simulink model "two_vehicle"  (R2020a)
settings: Solver=ode3  StartTime=0.0  StopTime=90  FixedStep=0.02  RelTol=1e-3  EnableMultiTasking=on
undefined symbols (not defined in the file): control, data
libraries: simulink_need_slupdate x10, simulink x2
settings Model: SimulationMode=accelerator  Creator=Owen  LastModifiedBy=rangeesh
settings DataIOCC: LimitDataPoints=on  SaveFormat=Array  ReturnWorkspaceOutputs=off
settings OptimizationCC: LifeSpan=inf  AccelVerboseBuild=on
settings DebuggingCC: SolverPrmCheckMsg=warning  SFUnexpectedBacktrackingDiag=warning  SFNoUnconditionalDefaultTransitionDiag=warning  SFExecutionAtInitializationDiag=none  ArithmeticOperatorsInVariantConditions=warning
settings HardwareCC: ProdBitPerPointer=32  ProdBitPerSizeT=32  ProdBitPerPtrDiffT=32  ProdLargestAtomicFloat=None  ProdIntDivRoundTo=Undefined  ProdEndianess=Unspecified  ProdWordSize=32  ProdHWDeviceType=32-bit Generic
settings ModelReferenceCC: PropagateSignalLabelsOutOfModel=off
settings SFSimCC: SimCustomInitializer=initTORCSLink();  SimCustomTerminator=terminateTORCSLink();  SimUserSources=TORCSLink.c  SimUserLibraries=librt.so  SimUseLocalCustomCode=off  SimParseCustomCode=off  SimBuildMode=sf_nonincremental_build  SimGenImportedTypeDefs=on  CustomCodeUndefinedFunction=UseInterfaceOnly
settings RTWCC: RTWUseLocalCustomCode=off
settings CodeAppCC: StateflowObjectComments=on
settings GRTTargetCC: TargetLangStandard=C89/C90 (ANSI)
settings ConfigComp: CovMetricSettings=dw  CovHtmlReporting=on  CovSaveCumulativeToWorkspaceVar=on  CovSaveSingleToWorkspaceVar=on  CovExternalEMLEnable=off  CovSFcnEnable=off

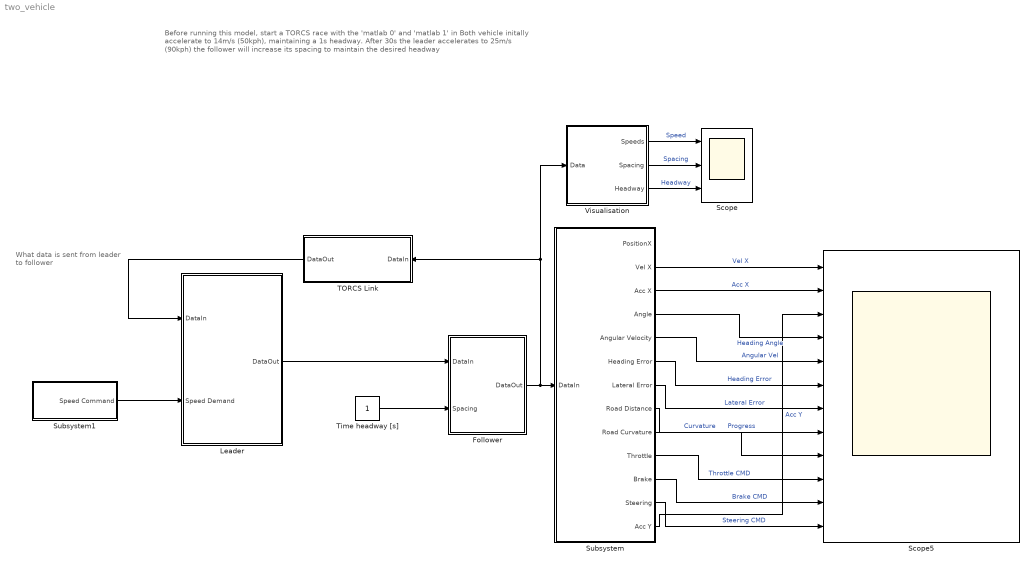
== system two_vehicle ==
  note: What data is sent from leader to follower
  note: Before running this model, start a TORCS race with the 'matlab 0' and 'matlab 1' in
      |
      | Both vehicle initally accelerate to 14m/s (50kph), maintaining a 1s headway.
      | After 30s the leader accelerates to 25m/s (90kph)
      | the follower will increase its spacing to maintain the desired headway
  Follower : Subsystem
      settings: CopyFcn=|
      | veh = str2num(get_param(gcb, 'vehicle'));
      | veh = veh + 1;
      | set_param(gcb,'vehicle',num2str(veh));
  Leader : Subsystem
  Scope : Scope  NumInputPorts=3
  Scope5 : Scope  NumInputPorts=12
  Subsystem : Subsystem
  Subsystem1 : Subsystem
  TORCS Link : Subsystem  LoadFcn=|  InitFcn=|
      LoadFcn=|
      | load VehicleBusses.mat;
      | src = 'TORCSLink.c';
      | init = 'initTORCSLink();';
      | term = 'terminateTORCSLink();';
      | simSrc = get_param(gcs,'SimUserSources');
      | simInit = get_param(gcs,'SimCustomInitializer');
      | simTerm = get_param(gcs,'SimCustomTerminator');
      | 
      | if isempty(strfind(simSrc,src))
      |   fprintf('Adding %s to Custom Sources\n', src);
      |   set_param(gcs,'SimUserSources', [simSrc 10 src]);
      | end
      | 
      | if isempty(strfind(simInit,init))
      |   fprintf('Adding %s to Custom Initialisation Code\n', init);
      |   set_param(gcs,'SimCustomInitializer', [simInit 10 init]);
      | end
      | 
      | if isempty(strfind(simTerm,term))
      |   fprintf('Adding %s to Custom Termination Code\n', term);
      |   set_param(gcs,'SimCustomTerminator', [simTerm 10 term]);
      | end
      | 
      | if isunix
      |     libs = 'librt.so';
      |     simLibs = get_param(gcs,'SimUserLibraries');
      | 
      |     if isempty(strfind(simLibs,libs))
      |       fprintf('Adding %s to Custom Libraries\n', libs);
      |       set_param(gcs,'SimUserLibraries', [simLibs 10 libs]);
      |     end
      | else
      |    set_param(gcs,'SimUserLibraries', '');
      | end
      | 
      | clear src init term simSrc simInit simTerm libs simLibs;
      InitFcn=|
      | load VehicleBusses.mat;
      | src = 'TORCSLink.c';
      | init = 'initTORCSLink();';
      | term = 'terminateTORCSLink();';
      | simSrc = get_param(gcs,'SimUserSources');
      | simInit = get_param(gcs,'SimCustomInitializer');
      | simTerm = get_param(gcs,'SimCustomTerminator');
      | 
      | if isempty(strfind(simSrc,src))
      |   fprintf('Adding %s to Custom Sources\n', src);
      |   set_param(gcs,'SimUserSources', [simSrc 10 src]);
      | end
      | 
      | if isempty(strfind(simInit,init))
      |   fprintf('Adding %s to Custom Initialisation Code\n', init);
      |   set_param(gcs,'SimCustomInitializer', [simInit 10 init]);
      | end
      | 
      | if isempty(strfind(simTerm,term))
      |   fprintf('Adding %s to Custom Termination Code\n', term);
      |   set_param(gcs,'SimCustomTerminator', [simTerm 10 term]);
      | end
      | 
      | if isunix
      |     libs = 'librt.so';
      |     simLibs = get_param(gcs,'SimUserLibraries');
      | 
      |     if isempty(strfind(simLibs,libs))
      |       fprintf('Adding %s to Custom Libraries\n', libs);
      |       set_param(gcs,'SimUserLibraries', [simLibs 10 libs]);
      |     end
      | else
      |    set_param(gcs,'SimUserLibraries', '');
      | end
      | 
      | clear src init term simSrc simInit simTerm libs simLibs;
  Time headway [s] : Constant
  Visualisation : Subsystem
  wires:
  Follower/1(DataOut) -> Visualisation/1(Data), TORCS Link/1(DataIn), Subsystem/1(DataIn)
  Leader/1(DataOut) -> Follower/1(DataIn)
  Time headway [s]/1 -> Follower/2(Spacing)
  Subsystem1/1(Speed Command) -> Leader/2(Speed Demand)
  Visualisation/2(Spacing) -> Scope/2  "Spacing"
  Visualisation/3(Headway) -> Scope/3  "Headway"
  Subsystem/2(Vel X) -> Scope5/1  "Vel X"
  Subsystem/3(Acc X) -> Scope5/2  "Acc X"
  Subsystem/11(Brake) -> Scope5/11  "Brake CMD"
  Subsystem/5(Angular Velocity) -> Scope5/5  "Angular Vel"
  Subsystem/10(Throttle) -> Scope5/10  "Throttle CMD"
  Visualisation/1(Speeds) -> Scope/1  "Speed"
  TORCS Link/1(DataOut) -> Leader/1(DataIn)
  Subsystem/12(Steering) -> Scope5/12  "Steering CMD"
  Subsystem/9(Road Curvature) -> Scope5/9  "Curvature"
  Subsystem/8(Road Distance) -> Scope5/8  "Progress"
  Subsystem/7(Lateral Error) -> Scope5/7  "Lateral Error"
  Subsystem/4(Angle) -> Scope5/4  "Heading Angle"
  Subsystem/6(Heading Error) -> Scope5/6  "Heading Error"
  Subsystem/13(Acc Y) -> Scope5/3  "Acc Y"

== system two_vehicle/Follower ==
  note: Use a Selector block to choose which vehicle data you want,
      | then use an Assignment to overwrite that vehicles data when you're done...
  DataIn : Inport
  Spacing : Inport  Port=2
  Assignment : Assignment  DiagnosticForDimensions=Warning  IndexOptions=Index vector (dialog)  Indices=2  OutputSizes=1
  Ego : Selector  InputPortWidth=10  IndexOptions=Index vector (dialog)  Indices=2  OutputSizes=1
  Follower Vehicle Control : Subsystem
  Leader : Selector  InputPortWidth=10  IndexOptions=Index vector (dialog)  Indices=1  OutputSizes=1
  DataOut : Outport
  wires:
  Ego/1 -> Follower Vehicle Control/3(Ego)
  DataIn/1 -> Ego/1, Leader/1, Assignment/1
  Assignment/1 -> DataOut/1
  Spacing/1 -> Follower Vehicle Control/1(Headway)
  Follower Vehicle Control/1(Data Out) -> Assignment/2
  Leader/1 -> Follower Vehicle Control/2(Leader)

== system two_vehicle/Leader ==
  note: Selector block is there to select which vehicle's
      | data you want to send
  note: Use a Selector block to choose which vehicle data you want,
      | then use an Assignment to overwrite that vehicles data when you're done...
  DataIn : Inport
  Speed Demand : Inport  Port=2
  Assignment : Assignment  DiagnosticForDimensions=Warning  IndexOptions=Index vector (dialog)  Indices=1  OutputSizes=1
  Lead Vehicle Control : Subsystem
  Selector : Selector  InputPortWidth=10  IndexOptions=Index vector (dialog)  Indices=1  OutputSizes=1
  DataOut : Outport
  wires:
  Speed Demand/1 -> Lead Vehicle Control/2(Speed Demand)
  DataIn/1 -> Selector/1, Assignment/1
  Selector/1 -> Lead Vehicle Control/1(Data In)
  Assignment/1 -> DataOut/1
  Lead Vehicle Control/1(Data Out) -> Assignment/2

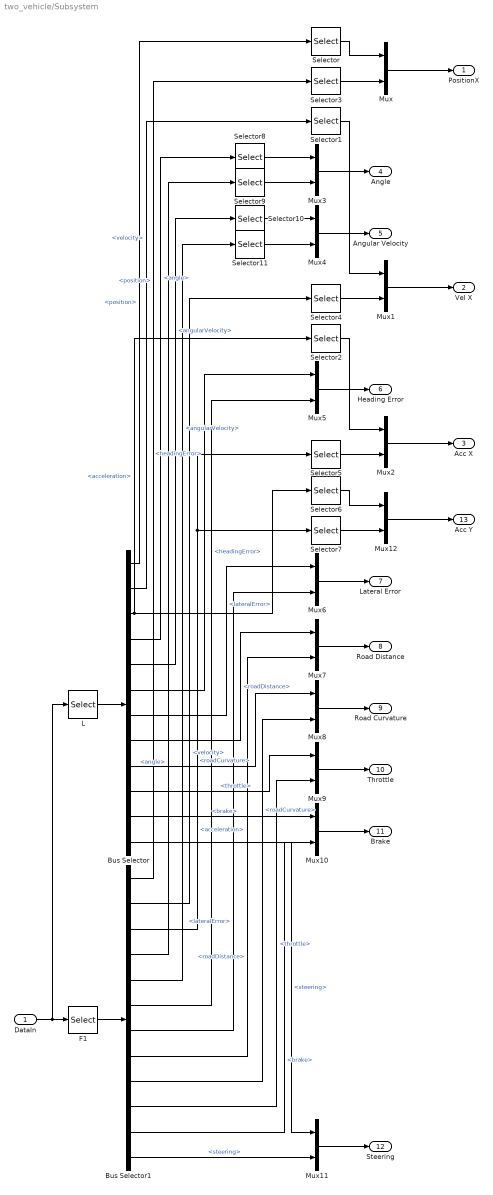
== system two_vehicle/Subsystem ==
  DataIn : Inport
  Bus Selector : BusSelector  OutputSignals=data.position,data.velocity,data.acceleration,data.angle,data.angularVelocity,data.headingError,data.lateralError,data.roadDistance,data.roadCurvature,control.throttle,control.brake,control.steering
  Bus Selector1 : BusSelector  OutputSignals=data.position,data.velocity,data.acceleration,data.angle,data.angularVelocity,data.headingError,data.lateralError,data.roadDistance,data.roadCurvature,control.throttle,control.brake,control.steering
  F1 : Selector  InputPortWidth=10  IndexOptions=Index vector (dialog)  Indices=2  OutputSizes=1
  L : Selector  InputPortWidth=10  IndexOptions=Index vector (dialog)  Indices=1  OutputSizes=1
  Mux{,1..12} (13 alike) : Mux  Inputs=2
  Selector{,1..5} (6 alike) : Selector  InputPortWidth=3  IndexOptions=Index vector (dialog)  Indices=1  OutputSizes=1
  Selector{8..11} (4 alike) : Selector  InputPortWidth=3  IndexOptions=Index vector (dialog)  Indices=3  OutputSizes=1
  Selector6 : Selector  InputPortWidth=3  IndexOptions=Index vector (dialog)  Indices=2  OutputSizes=1
  Selector7 : Selector  InputPortWidth=3  IndexOptions=Index vector (dialog)  Indices=2  OutputSizes=1
  PositionX : Outport
  Vel X : Outport  Port=2
  Acc X : Outport  Port=3
  Angle : Outport  Port=4
  Angular Velocity : Outport  Port=5
  Heading Error : Outport  Port=6
  Lateral Error : Outport  Port=7
  Road Distance : Outport  Port=8
  Road Curvature : Outport  Port=9
  Throttle : Outport  Port=10
  Brake : Outport  Port=11
  Steering : Outport  Port=12
  Acc Y : Outport  Port=13
  wires:
  Bus Selector/3 -> Selector6/1, Selector2/1  "<acceleration>"
  DataIn/1 -> F1/1, L/1
  Selector6/1 -> Mux12/1
  Mux7/1 -> Road Distance/1
  Bus Selector/11 -> Mux10/1  "<brake>"
  Bus Selector/6 -> Mux5/1  "<headingError>"
  Bus Selector/4 -> Selector8/1  "<angle>"
  Bus Selector/5 -> Selector10/1  "<angularVelocity>"
  Bus Selector1/5 -> Selector11/1  "<angularVelocity>"
  Mux4/1 -> Angular Velocity/1
  Mux9/1 -> Throttle/1
  Mux1/1 -> Vel X/1
  Mux6/1 -> Lateral Error/1
  Bus Selector1/7 -> Mux6/2  "<lateralError>"
  Selector/1 -> Mux/1
  Bus Selector1/3 -> Selector7/1, Selector5/1  "<acceleration>"
  Bus Selector1/12 -> Mux11/2  "<steering>"
  Selector3/1 -> Mux/2
  Selector4/1 -> Mux1/2
  Mux5/1 -> Heading Error/1
  Mux10/1 -> Brake/1
  Bus Selector1/9 -> Mux8/2  "<roadCurvature>"
  Mux8/1 -> Road Curvature/1
  Bus Selector/12 -> Mux11/1  "<steering>"
  F1/1 -> Bus Selector1/1
  Bus Selector1/10 -> Mux9/2  "<throttle>"
  Mux/1 -> PositionX/1
  Mux11/1 -> Steering/1
  Bus Selector1/11 -> Mux10/2  "<brake>"
  Bus Selector/10 -> Mux9/1  "<throttle>"
  Bus Selector/7 -> Mux6/1  "<lateralError>"
  Bus Selector/9 -> Mux8/1  "<roadCurvature>"
  Bus Selector1/2 -> Selector4/1  "<velocity>"
  Bus Selector1/1 -> Selector3/1  "<position>"
  Mux12/1 -> Acc Y/1
  Bus Selector1/4 -> Selector9/1  "<angle>"
  Bus Selector1/6 -> Mux5/2  "<headingError>"
  Selector7/1 -> Mux12/2
  Selector2/1 -> Mux2/1
  L/1 -> Bus Selector/1
  Bus Selector/2 -> Selector1/1  "<velocity>"
  Selector1/1 -> Mux1/1
  Bus Selector1/8 -> Mux7/2  "<roadDistance>"
  Mux2/1 -> Acc X/1
  Bus Selector/1 -> Selector/1  "<position>"
  Bus Selector/8 -> Mux7/1  "<roadDistance>"
  Selector5/1 -> Mux2/2
  Mux3/1 -> Angle/1
  Selector8/1 -> Mux3/1
  Selector9/1 -> Mux3/2
  Selector10/1 -> Mux4/1
  Selector11/1 -> Mux4/2

== system two_vehicle/Subsystem1 ==
  Clock : Clock
  Constant : Constant  Value=[14, 25, 0]
  Index Selector : MATLAB Function  TreatAsAtomicUnit=on
  Selector : Selector  InputPortWidth=3  IndexOptions=Index vector (port)  Indices=[1 3]  OutputSizes=1
  Speed Command : Outport
  wires:
  Clock/1 -> Index Selector/1(time)
  Index Selector/1(speed_command_index) -> Selector/2
  Constant/1 -> Selector/1
  Selector/1 -> Speed Command/1

== system two_vehicle/TORCS Link ==
  note: This subsystem handles the communicatrion with TORCS via a MATLAB function.
      | The simulation must be configured to run at a fixed sample time equal to the rate at which TORCS updates its robots (0.02s by default)
      | Data returned from TORCS is passed through a First-Order-Hold to allow continuous design in Simulink
      | Data for a maximum of 10 vehicles is returned, but not all vehicles need be present in the race
  DataIn : Inport
  FOHs : Subsystem  TreatAsAtomicUnit=on
  Memory : Memory
  Stop Simulation : Stop
  TORCSLink : MATLAB Function  TreatAsAtomicUnit=on
  DataOut : Outport
  wires:
  Memory/1 -> TORCSLink/1(vehicleDataIn)
  TORCSLink/1(vehicleDataOut) -> FOHs/1(In1)
  FOHs/1(Out1) -> DataOut/1
  DataIn/1 -> Memory/1
  TORCSLink/2(stop) -> Stop Simulation/1

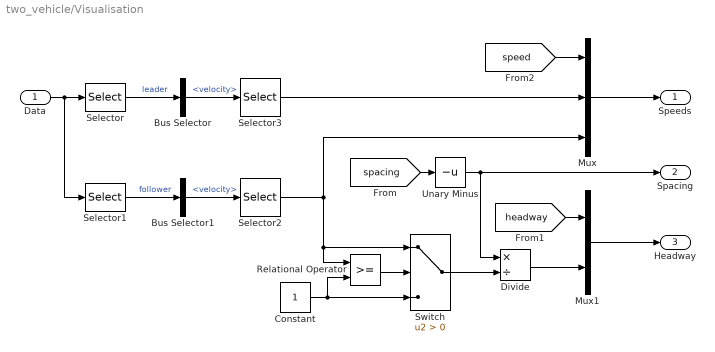
== system two_vehicle/Visualisation ==
  Data : Inport
  Bus Selector : BusSelector  OutputSignals=data.velocity
  Bus Selector1 : BusSelector  OutputSignals=data.velocity
  Constant : Constant
  Divide : Product  Inputs=*/
  Mux : Mux  Inputs=3
  Mux1 : Mux  Inputs=2
  Relational Operator : RelationalOperator  OutDataTypeStr=boolean  RndMeth=Nearest
  Selector : Selector  InputPortWidth=10  IndexOptions=Index vector (dialog)  Indices=1  OutputSizes=1
  Selector1 : Selector  InputPortWidth=10  IndexOptions=Index vector (dialog)  Indices=2  OutputSizes=1
  Selector2 : Selector  InputPortWidth=3  IndexOptions=Index vector (dialog)  Indices=1  OutputSizes=1
  Selector3 : Selector  InputPortWidth=3  IndexOptions=Index vector (dialog)  Indices=1  OutputSizes=1
  Switch : Switch  Criteria=u2 > Threshold
  Unary Minus : UnaryMinus
  Speeds : Outport
  Spacing : Outport  Port=2
  Headway : Outport  Port=3
  wires:
  Data/1 -> Selector1/1, Selector/1
  Selector/1 -> Bus Selector/1  "leader"
  Selector1/1 -> Bus Selector1/1  "follower"
  Bus Selector1/1 -> Selector2/1  "<velocity>"
  Bus Selector/1 -> Selector3/1  "<velocity>"
  Selector3/1 -> Mux/2
  Selector2/1 -> Relational Operator/1, Switch/1, Mux/3
  Mux/1 -> Speeds/1
  [spacing] -> Unary Minus/1
  Unary Minus/1 -> Divide/1, Spacing/1
  [speed] -> Mux/1
  Mux1/1 -> Headway/1
  Divide/1 -> Mux1/2
  [headway] -> Mux1/1
  Switch/1 -> Divide/2
  Relational Operator/1 -> Switch/2
  Constant/1 -> Switch/3, Relational Operator/2

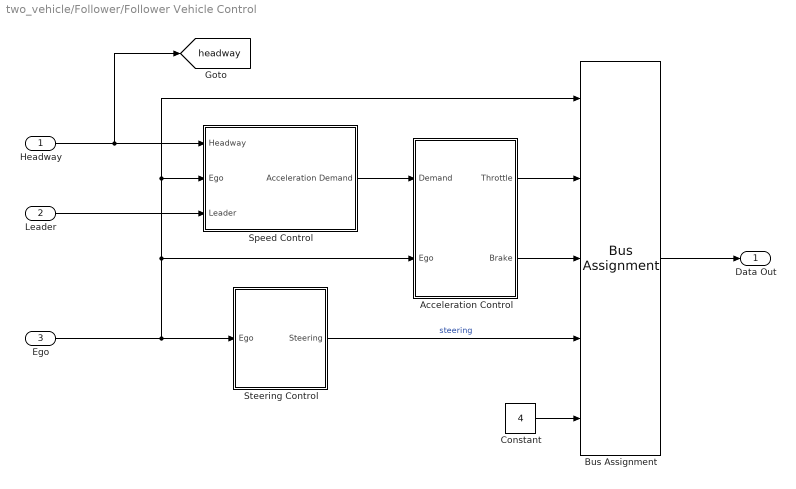
== system two_vehicle/Follower/Follower Vehicle Control ==
  Headway : Inport
  Leader : Inport  Port=2
  Ego : Inport  Port=3
  Acceleration Control : Subsystem
  Bus Assignment : BusAssignment  AssignedSignals=control.throttle,control.brake,control.steering,control.gear
  Constant : Constant  Value=4  OutDataTypeStr=int32
  Speed Control : Subsystem
  Steering Control : Subsystem
  Data Out : Outport
  tag scope: headway=global
  wires:
  Bus Assignment/1 -> Data Out/1
  Speed Control/1(Acceleration Demand) -> Acceleration Control/1(Demand)
  Headway/1 -> [headway], Speed Control/1(Headway)
  Ego/1 -> Bus Assignment/1, Speed Control/2(Ego), Acceleration Control/2(Ego), Steering Control/1(Ego)
  Leader/1 -> Speed Control/3(Leader)
  Acceleration Control/2(Brake) -> Bus Assignment/3
  Acceleration Control/1(Throttle) -> Bus Assignment/2
  Steering Control/1(Steering) -> Bus Assignment/4  "steering"
  Constant/1 -> Bus Assignment/5

== system two_vehicle/Leader/Lead Vehicle Control ==
  Data In : Inport
  Speed Demand : Inport  Port=2
  Acceleration Control : Subsystem
  Bus Assignment : BusAssignment  AssignedSignals=control.throttle,control.brake,control.steering,control.gear
  Constant : Constant  Value=4  OutDataTypeStr=int32
  Speed Control : Subsystem
  Steering Control : Subsystem
  Data Out : Outport
  tag scope: speed=global
  wires:
  Speed Demand/1 -> [speed], Speed Control/1(Demand)
  Bus Assignment/1 -> Data Out/1
  Speed Control/1(Acceleration Demand) -> Acceleration Control/1(Demand)
  Data In/1 -> Steering Control/1(Ego), Speed Control/2(Velocity), Bus Assignment/1, Acceleration Control/2(Ego)
  Acceleration Control/2(Brake) -> Bus Assignment/3
  Acceleration Control/1(Throttle) -> Bus Assignment/2
  Steering Control/1(Steering) -> Bus Assignment/4
  Constant/1 -> Bus Assignment/5

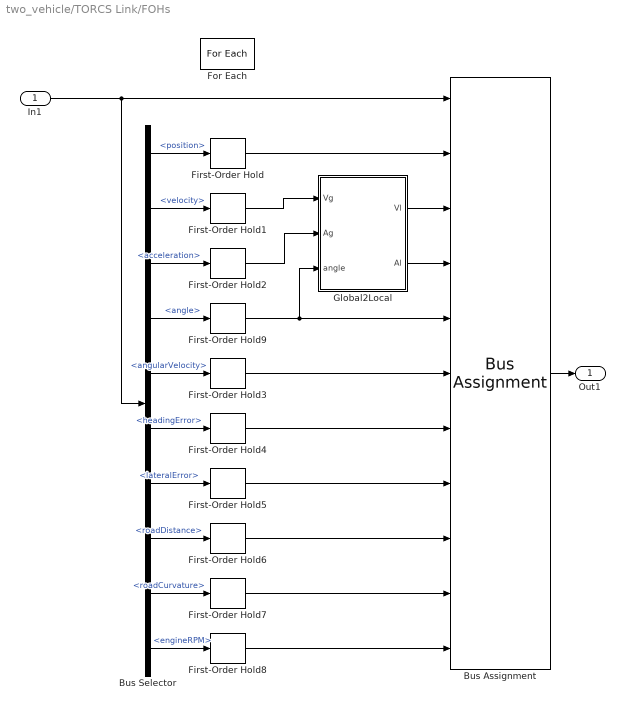
== system two_vehicle/TORCS Link/FOHs ==
  In1 : Inport  Partition=on  PartitionDimension=1  PartitionWidth=1  PartitionOffset=0
  Bus Assignment : BusAssignment  AssignedSignals=data.position,data.velocity,data.acceleration,data.angle,data.angularVelocity,data.headingError,data.lateralError,data.roadDistance,data.roadCurvature,data.engineRPM
  Bus Selector : BusSelector  OutputSignals=data.position,data.velocity,data.acceleration,data.angle,data.angularVelocity,data.headingError,data.lateralError,data.roadDistance,data.roadCurvature,data.engineRPM
  First-Order Hold{,1..9} (10 alike) : simulink_need_slupdate/First-Order Hold  DisableCoverage=on  Ts=0.02
      settings: SourceProductBaseCode=SL
  For Each : ForEach  DisableCoverage=on
  Global2Local : MATLAB Function  TreatAsAtomicUnit=on
  Out1 : Outport  ConcatenationDimension=1
  wires:
  Bus Assignment/1 -> Out1/1
  Bus Selector/10 -> First-Order Hold8/1  "<engineRPM>"
  Bus Selector/9 -> First-Order Hold7/1  "<roadCurvature>"
  Bus Selector/8 -> First-Order Hold6/1  "<roadDistance>"
  Bus Selector/7 -> First-Order Hold5/1  "<lateralError>"
  Bus Selector/6 -> First-Order Hold4/1  "<headingError>"
  Bus Selector/5 -> First-Order Hold3/1  "<angularVelocity>"
  Bus Selector/3 -> First-Order Hold2/1  "<acceleration>"
  Bus Selector/2 -> First-Order Hold1/1  "<velocity>"
  Bus Selector/1 -> First-Order Hold/1  "<position>"
  In1/1 -> Bus Assignment/1, Bus Selector/1
  Bus Selector/4 -> First-Order Hold9/1  "<angle>"
  First-Order Hold9/1 -> Global2Local/3(angle), Bus Assignment/5
  First-Order Hold3/1 -> Bus Assignment/6
  First-Order Hold4/1 -> Bus Assignment/7
  First-Order Hold5/1 -> Bus Assignment/8
  First-Order Hold6/1 -> Bus Assignment/9
  First-Order Hold7/1 -> Bus Assignment/10
  First-Order Hold8/1 -> Bus Assignment/11
  First-Order Hold1/1 -> Global2Local/1(Vg)
  First-Order Hold2/1 -> Global2Local/2(Ag)
  First-Order Hold/1 -> Bus Assignment/2
  Global2Local/2(Al) -> Bus Assignment/4
  Global2Local/1(Vl) -> Bus Assignment/3

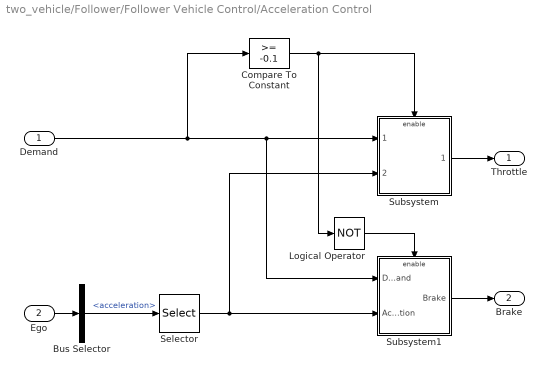
== system two_vehicle/Follower/Follower Vehicle Control/Acceleration Control ==
  Demand : Inport
  Ego : Inport  Port=2
  Bus Selector : BusSelector  OutputSignals=data.acceleration
  Compare To Constant : simulink/Logic and Bit Operations/Compare To Constant  relop=>=  const=-0.1  OutDataTypeStr=boolean
  Logical Operator : Logic  Operator=NOT  AllPortsSameDT=off  OutDataTypeStr=boolean
  Selector : Selector  InputPortWidth=3  IndexOptions=Index vector (dialog)  Indices=1  OutputSizes=1
  Subsystem : Subsystem
  Subsystem1 : Subsystem
  Throttle : Outport
  Brake : Outport  Port=2
  wires:
  Selector/1 -> Subsystem/2(Acceleration), Subsystem1/2(Acceleration)
  Demand/1 -> Compare To Constant/1, Subsystem1/1(Demand), Subsystem/1(Demand)
  Subsystem1/1(Brake) -> Brake/1
  Subsystem/1(Throttle) -> Throttle/1
  Compare To Constant/1 -> Subsystem/Enable, Logical Operator/1
  Logical Operator/1 -> Subsystem1/Enable
  Ego/1 -> Bus Selector/1
  Bus Selector/1 -> Selector/1  "<acceleration>"

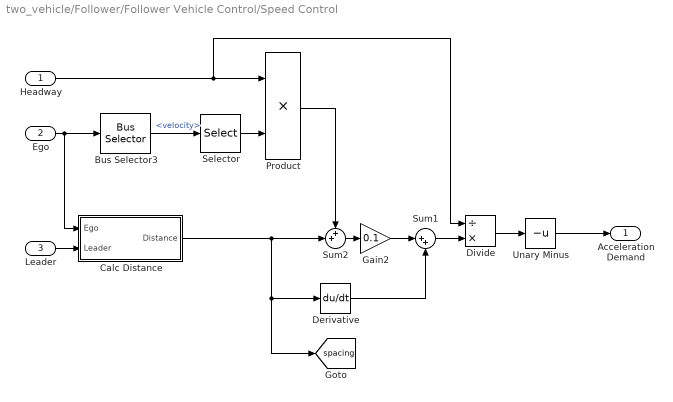
== system two_vehicle/Follower/Follower Vehicle Control/Speed Control ==
  Headway : Inport
  Ego : Inport  Port=2
  Leader : Inport  Port=3
  Bus Selector3 : BusSelector  OutputSignals=data.velocity
  Calc Distance : Subsystem
  Derivative : Derivative
  Divide : Product  Inputs=/*
  Gain2 : Gain  Gain=0.1
  Product : Product
  Selector : Selector  InputPortWidth=3  IndexOptions=Index vector (dialog)  Indices=1  OutputSizes=1
  Sum1 : Sum  Inputs=|++
  Sum2 : Sum  Inputs=++|
  Unary Minus : UnaryMinus
  Acceleration Demand : Outport
  tag scope: spacing=global
  wires:
  Ego/1 -> Calc Distance/1(Ego), Bus Selector3/1
  Leader/1 -> Calc Distance/2(Leader)
  Bus Selector3/1 -> Selector/1  "<velocity>"
  Headway/1 -> Divide/1, Product/1
  Selector/1 -> Product/2
  Calc Distance/1(Distance) -> Derivative/1, [spacing], Sum2/2
  Product/1 -> Sum2/1
  Sum2/1 -> Gain2/1
  Gain2/1 -> Sum1/1
  Derivative/1 -> Sum1/2
  Sum1/1 -> Divide/2
  Divide/1 -> Unary Minus/1
  Unary Minus/1 -> Acceleration Demand/1

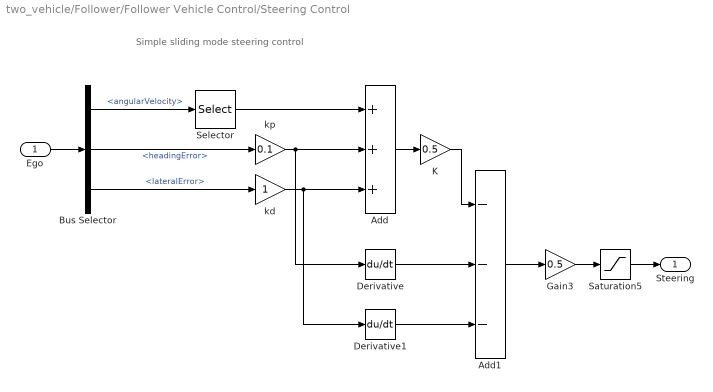
== system two_vehicle/Follower/Follower Vehicle Control/Steering Control ==
  note: Simple sliding mode steering control
  Ego : Inport
  Add : Sum  Inputs=+++
  Add1 : Sum  Inputs=---
  Bus Selector : BusSelector  OutputSignals=data.angularVelocity,data.headingError,data.lateralError
  Derivative : Derivative
  Derivative1 : Derivative
  Gain3 : Gain  Gain=0.5
  K : Gain  Gain=0.5
  Saturation5 : Saturate
  Selector : Selector  InputPortWidth=3  IndexOptions=Index vector (dialog)  Indices=3  OutputSizes=1
  kd : Gain
  kp : Gain  Gain=0.1
  Steering : Outport
  wires:
  Ego/1 -> Bus Selector/1
  Add1/1 -> Gain3/1
  K/1 -> Add1/1
  Derivative1/1 -> Add1/3
  Derivative/1 -> Add1/2
  Add/1 -> K/1
  kp/1 -> Derivative/1, Add/2
  kd/1 -> Derivative1/1, Add/3
  Bus Selector/3 -> kd/1  "<lateralError>"
  Bus Selector/2 -> kp/1  "<headingError>"
  Gain3/1 -> Saturation5/1
  Saturation5/1 -> Steering/1
  Selector/1 -> Add/1
  Bus Selector/1 -> Selector/1  "<angularVelocity>"

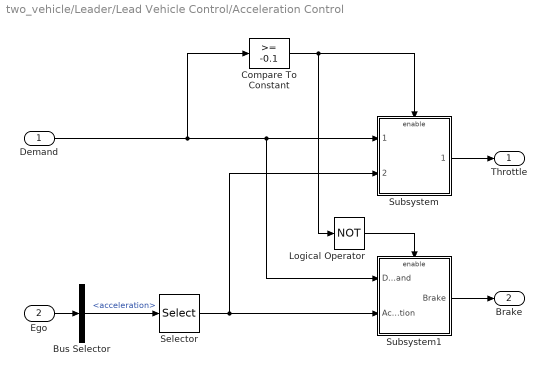
== system two_vehicle/Leader/Lead Vehicle Control/Acceleration Control ==
  Demand : Inport
  Ego : Inport  Port=2
  Bus Selector : BusSelector  OutputSignals=data.acceleration
  Compare To Constant : simulink/Logic and Bit Operations/Compare To Constant  relop=>=  const=-0.1  OutDataTypeStr=boolean
  Logical Operator : Logic  Operator=NOT  AllPortsSameDT=off  OutDataTypeStr=boolean
  Selector : Selector  InputPortWidth=3  IndexOptions=Index vector (dialog)  Indices=1  OutputSizes=1
  Subsystem : Subsystem
  Subsystem1 : Subsystem
  Throttle : Outport
  Brake : Outport  Port=2
  wires:
  Selector/1 -> Subsystem/2(Acceleration), Subsystem1/2(Acceleration)
  Demand/1 -> Compare To Constant/1, Subsystem1/1(Demand), Subsystem/1(Demand)
  Subsystem1/1(Brake) -> Brake/1
  Subsystem/1(Throttle) -> Throttle/1
  Compare To Constant/1 -> Subsystem/Enable, Logical Operator/1
  Logical Operator/1 -> Subsystem1/Enable
  Ego/1 -> Bus Selector/1
  Bus Selector/1 -> Selector/1  "<acceleration>"

== system two_vehicle/Leader/Lead Vehicle Control/Speed Control ==
  Demand : Inport
  Velocity : Inport  Port=2
  Bus Selector : BusSelector  OutputSignals=data.velocity
  Gain : Gain  Gain=0.5
  Rate Limiter : RateLimiter  RisingSlewLimit=inf  FallingSlewLimit=-inf  SampleTimeMode=inherited
  Saturation : Saturate  UpperLimit=2  LowerLimit=-4
  Selector : Selector  InputPortWidth=3  IndexOptions=Index vector (dialog)  Indices=1  OutputSizes=1
  Sum : Sum  Inputs=|+-
  Acceleration Demand : Outport
  wires:
  Gain/1 -> Saturation/1
  Sum/1 -> Gain/1
  Demand/1 -> Sum/1
  Saturation/1 -> Rate Limiter/1
  Selector/1 -> Sum/2
  Rate Limiter/1 -> Acceleration Demand/1
  Velocity/1 -> Bus Selector/1
  Bus Selector/1 -> Selector/1  "<velocity>"

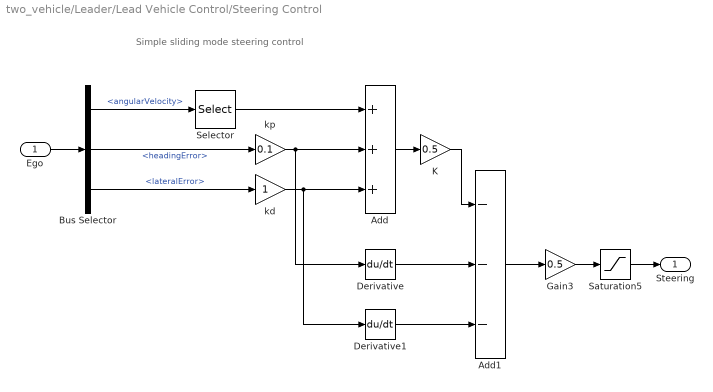
== system two_vehicle/Leader/Lead Vehicle Control/Steering Control ==
  note: Simple sliding mode steering control
  Ego : Inport
  Add : Sum  Inputs=+++
  Add1 : Sum  Inputs=---
  Bus Selector : BusSelector  OutputSignals=data.angularVelocity,data.headingError,data.lateralError
  Derivative : Derivative
  Derivative1 : Derivative
  Gain3 : Gain  Gain=0.5
  K : Gain  Gain=0.5
  Saturation5 : Saturate
  Selector : Selector  InputPortWidth=3  IndexOptions=Index vector (dialog)  Indices=3  OutputSizes=1
  kd : Gain
  kp : Gain  Gain=0.1
  Steering : Outport
  wires:
  Ego/1 -> Bus Selector/1
  Add1/1 -> Gain3/1
  K/1 -> Add1/1
  Derivative1/1 -> Add1/3
  Derivative/1 -> Add1/2
  Add/1 -> K/1
  kp/1 -> Derivative/1, Add/2
  kd/1 -> Derivative1/1, Add/3
  Bus Selector/3 -> kd/1  "<lateralError>"
  Bus Selector/2 -> kp/1  "<headingError>"
  Gain3/1 -> Saturation5/1
  Saturation5/1 -> Steering/1
  Selector/1 -> Add/1
  Bus Selector/1 -> Selector/1  "<angularVelocity>"

== system two_vehicle/Follower/Follower Vehicle Control/Acceleration Control/Subsystem ==
  Demand : Inport
  Acceleration : Inport  Port=2
  Enable : EnablePort  StatesWhenEnabling=reset
  Gain : Gain  Gain=1.5
  Gain1 : Gain  Gain=10
  Integrator Limited : Integrator  LimitOutput=on  UpperSaturationLimit=1  LowerSaturationLimit=-1
  Sum : Sum  Inputs=++|
  Sum1 : Sum  Inputs=+-|
  Throttle : Outport  OutputWhenDisabled=reset  InitialOutput=0
  wires:
  Gain/1 -> Sum/1
  Integrator Limited/1 -> Sum/2
  Gain1/1 -> Integrator Limited/1
  Sum/1 -> Throttle/1
  Demand/1 -> Sum1/1, Gain/1
  Acceleration/1 -> Sum1/2
  Sum1/1 -> Gain1/1

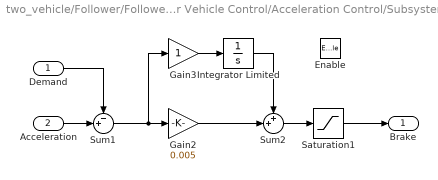
== system two_vehicle/Follower/Follower Vehicle Control/Acceleration Control/Subsystem1 ==
  Demand : Inport
  Acceleration : Inport  Port=2
  Enable : EnablePort  StatesWhenEnabling=reset
  Gain2 : Gain  Gain=0.005
  Gain3 : Gain
  Integrator Limited : Integrator  LimitOutput=on  UpperSaturationLimit=1  LowerSaturationLimit=-1
  Saturation1 : Saturate  UpperLimit=1  LowerLimit=0
  Sum1 : Sum  Inputs=-+|
  Sum2 : Sum  Inputs=++|
  Brake : Outport  OutputWhenDisabled=reset  InitialOutput=0
  wires:
  Saturation1/1 -> Brake/1
  Sum2/1 -> Saturation1/1
  Gain2/1 -> Sum2/2
  Integrator Limited/1 -> Sum2/1
  Gain3/1 -> Integrator Limited/1
  Sum1/1 -> Gain2/1, Gain3/1
  Demand/1 -> Sum1/1
  Acceleration/1 -> Sum1/2

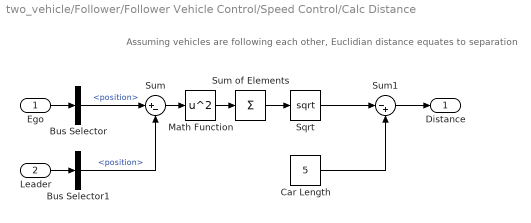
== system two_vehicle/Follower/Follower Vehicle Control/Speed Control/Calc Distance ==
  note: Assuming vehicles are following each other, Euclidian distance equates to separation
  Ego : Inport
  Leader : Inport  Port=2
  Bus Selector : BusSelector  OutputSignals=data.position
  Bus Selector1 : BusSelector  OutputSignals=data.position
  Car Length : Constant  Value=5
  Math Function : Math  Operator=square  SignedPower=on  SaturateOnIntegerOverflow=on
  Sqrt : Sqrt  SaturateOnIntegerOverflow=on
  Sum : Sum  Inputs=|+-
  Sum of Elements : Sum  Inputs=+
  Sum1 : Sum  Inputs=|-+
  Distance : Outport
  wires:
  Ego/1 -> Bus Selector/1
  Leader/1 -> Bus Selector1/1
  Bus Selector/1 -> Sum/1  "<position>"
  Bus Selector1/1 -> Sum/2  "<position>"
  Sum/1 -> Math Function/1
  Math Function/1 -> Sum of Elements/1
  Sum of Elements/1 -> Sqrt/1
  Sum1/1 -> Distance/1
  Sqrt/1 -> Sum1/1
  Car Length/1 -> Sum1/2

== system two_vehicle/Leader/Lead Vehicle Control/Acceleration Control/Subsystem ==
  note: Throttle = Demand*1.5 + Integral Error*10?
  Demand : Inport
  Acceleration : Inport  Port=2
  Enable : EnablePort  StatesWhenEnabling=reset
  Gain : Gain  Gain=1.5
  Gain1 : Gain  Gain=10
  Integrator Limited : Integrator  LimitOutput=on  UpperSaturationLimit=1  LowerSaturationLimit=-1
  Sum : Sum  Inputs=++|
  Sum1 : Sum  Inputs=+-|
  Throttle : Outport  OutputWhenDisabled=reset  InitialOutput=0
  wires:
  Gain/1 -> Sum/1
  Integrator Limited/1 -> Sum/2
  Gain1/1 -> Integrator Limited/1
  Sum/1 -> Throttle/1
  Demand/1 -> Sum1/1, Gain/1
  Acceleration/1 -> Sum1/2
  Sum1/1 -> Gain1/1

== system two_vehicle/Leader/Lead Vehicle Control/Acceleration Control/Subsystem1 ==
  note: Error*0.005 + Integral Error * 1
  Demand : Inport
  Acceleration : Inport  Port=2
  Enable : EnablePort  StatesWhenEnabling=reset
  Gain2 : Gain  Gain=0.005
  Gain3 : Gain
  Integrator Limited : Integrator  LimitOutput=on  UpperSaturationLimit=1  LowerSaturationLimit=-1
  Saturation1 : Saturate  UpperLimit=1  LowerLimit=0
  Sum1 : Sum  Inputs=-+|
  Sum2 : Sum  Inputs=++|
  Brake : Outport  OutputWhenDisabled=reset  InitialOutput=0
  wires:
  Saturation1/1 -> Brake/1
  Sum2/1 -> Saturation1/1
  Gain2/1 -> Sum2/2
  Integrator Limited/1 -> Sum2/1
  Gain3/1 -> Integrator Limited/1
  Sum1/1 -> Gain2/1, Gain3/1
  Demand/1 -> Sum1/1
  Acceleration/1 -> Sum1/2

== matlab function two_vehicle/TORCS Link/TORCSLink ==
  data: vehicleDataIn input Bus: VehicleBus size=10; vehicleDataOut output Bus: VehicleBus size=10; stop output
function [vehicleDataOut, stop] = TORCSLink(vehicleDataIn)
%#codegen
stop = 0;
flag = int32(0);

% Simulink doesn't like passing the array of structures to C function (no
% idea why?!), so we have to seperate out the three stages

% Update vehicle control values in TORCS
for i=1:10
    flag = coder.ceval('setVehicleControl', int32(i-1), vehicleDataIn(i).control);
    if (flag < 0)
        fprintf('No connection to TORCS!\n');
        stop = 1;
    end
end

% Tell TORCS it can update (this function hangs until new data is
% available)
flag = coder.ceval('updateTORCS');
if (flag < 0)
    fprintf('No data from TORCS! (%d) \n', flag);
    stop = 1;
end

% Read in new data from TORCS
for i=1:10
    % Can't pass this directly to coder.ref
    data = vehicleDataIn(i).data;
    flag = coder.ceval('getVehicleData', int32(i-1), coder.ref(data));
    vehicleDataIn(i).data = data;
    if (flag < 0)
        fprintf('No connection to TORCS!\n');
        stop = 1;
    end
end

vehicleDataOut = vehicleDataIn;

== matlab function two_vehicle/TORCS Link/FOHs/Global2Local ==
  data: Vg input; Ag input; angle input; Vl output; Al output
function [Vl,Al] = fcn(Vg,Ag,angle)
%#codegen

phi=angle(3);
R = [cos(phi) sin(phi) 0; -sin(phi) cos(phi) 0; 0 0 1];

Vl = R*Vg;
Al = R*Ag;

== matlab function two_vehicle/Subsystem1/Index Selector ==
  data: time input; speed_command_index output
function speed_command_index = fcn(time)

if time < 5
    speed_command_index = 1;
elseif time>=5 && time<30
    speed_command_index = 2;
elseif time>=30 && time<85
    speed_command_index = 3;
else
    speed_command_index = 4;
end
